simulink model "Quad_F450_Model"  (R2023a)
settings: Solver=FixedStepAuto  StartTime=0.0  StopTime=inf  FixedStep=Copter.SimTs  RelTol=1e-3
InitFcn:
  | load("motor_data.mat")
  | run("Parameters.m")
undefined symbols (not defined in the file or in its folder): Controller, Copter, DiscIntNeverNeededParam, Earth, init, Keyboard, motor_data, w_der_filt, WGS84
libraries: sharedutil x12, slpidlib x8, sharedtransform x5, aerolibpropulsionsys x4, simulink_extras x3, matrix_library x3, shared6dof x1, aerolibtransform2 x1, aerolibatmos2 x1, aerolibsim3d x1, sim3dlib x1
(part 3 of 3)

== system Quad_F450_Model/DYNAMIC_MODEL/Motor Forces and Moments/Motor 4/Moments ==
  rho : Inport
  w : Inport  Port=2
  Arm : Inport  Port=3
  Abs1 : Abs  SaturateOnIntegerOverflow=off
  Bus Selector : BusSelector  OutputSignals=prop4_cq,prop4_radius_m
  Constant : Constant  Value=pi
  Gain : Gain  Gain=-1
  Mxy : Constant  Value=[0 0]
  Product : Product  Inputs=5
  Product1 : Product
  Product5 : Product
  Product7 : Product
  Square : Math  Operator=square
  Vector Concatenate3 : Concatenate
  Mxyz : Outport
  wires:
  Product1/1 -> Product7/2
  Mxy/1 -> Vector Concatenate3/1
  rho/1 -> Product7/1
  Product7/1 -> Vector Concatenate3/2
  Abs1/1 -> Product5/2
  w/1 -> Abs1/1, Product5/1
  Vector Concatenate3/1 -> Mxyz/1
  [CQ] -> Product/1
  Constant/1 -> Product/2
  [R] -> Product/5, Square/1
  Square/1 -> Product/3, Product/4
  Product/1 -> Gain/1
  Product5/1 -> Product1/1
  Gain/1 -> [d_rads]
  [d_rads] -> Product1/2
  Arm/1 -> Bus Selector/1
  Bus Selector/1 -> [CQ]  "<prop4_cq>"
  Bus Selector/2 -> [R]  "<prop4_radius_m>"

== system Quad_F450_Model/DYNAMIC_MODEL/Motor Forces and Moments/Motor 4/Subsystem ==
  Vb : Inport
  pqr : Inport  Port=2
  w : Inport  Port=3
  Arm : Inport  Port=4
  3x3 Cross Product : sharedutil/3x3 Cross Product  aMode=aMode
  Add : Sum
  Bus Selector : BusSelector  OutputSignals=cg2motor_arm4_m
  Demux : Demux  Outputs=2
  Gain : Gain  Gain=Copter.blade_flap_active
  J : Subsystem
  Sum : aerolibpropulsionsys/Flap/Sum  Inputs=++|  CollapseDim=1  OutMin=[]  OutMax=[]  SampleTime=-1
  beta1 : Subsystem
  beta2 : Subsystem
  lc and mu : Subsystem
  a1s : Outport
  b1s : Outport  Port=2
  wires:
  w/1 -> beta2/2(w), beta1/4(w), lc and mu/2(w)
  Sum/1 -> lc and mu/1(Vr), J/1(Vr)  "Vr"
  Demux/1 -> a1s/1
  beta1/1(beta1) -> Add/1
  Add/1 -> Gain/1  "beta"
  pqr/1 -> beta2/3(pqr), 3x3 Cross Product/1
  beta2/1(beta2) -> Add/2
  Arm/1 -> Bus Selector/1, beta1/5(Arm), beta2/4(Arm), lc and mu/3(Arm)
  lc and mu/2(mu) -> beta2/1(mu), beta1/3(mu)
  lc and mu/1(lc) -> beta1/2(lc)
  Demux/2 -> b1s/1
  3x3 Cross Product/1 -> Sum/2
  Vb/1 -> Sum/1
  Bus Selector/1 -> 3x3 Cross Product/2  "<cg2motor_arm4_m>"
  J/1(J) -> beta1/1(J)
  Gain/1 -> Demux/1

== system Quad_F450_Model/DYNAMIC_MODEL/Motor Forces and Moments/Motor 1/Subsystem/J ==
  Vr : Inport
  Gain : Gain  Gain=-1
  Matrix Concatenate : Concatenate  Mode=Multidimensional array  ConcatenateDimension=2
  Selector2 : Selector  InputPortWidth=3  IndexOptions=Index vector (dialog)  Indices=[2]  OutputSizes=1
  Selector3 : Selector  InputPortWidth=3  IndexOptions=Index vector (dialog)  Indices=[1]  OutputSizes=1
  Trigonometric Function1 : Trigonometry  Operator=atan2
  Trigonometric Function2 : Trigonometry  Operator=sincos
  Vector Concatenate : Concatenate
  Vector Concatenate1 : Concatenate
  J : Outport
  wires:
  Vr/1 -> Selector2/1, Selector3/1
  Vector Concatenate/1 -> Matrix Concatenate/1
  Matrix Concatenate/1 -> J/1  "J"
  Trigonometric Function2/1 -> Gain/1, Vector Concatenate/2
  Trigonometric Function1/1 -> Trigonometric Function2/1  "j"
  Selector2/1 -> Trigonometric Function1/1
  Gain/1 -> Vector Concatenate1/1
  Selector3/1 -> Trigonometric Function1/2
  Trigonometric Function2/2 -> Vector Concatenate1/2, Vector Concatenate/1
  Vector Concatenate1/1 -> Matrix Concatenate/2

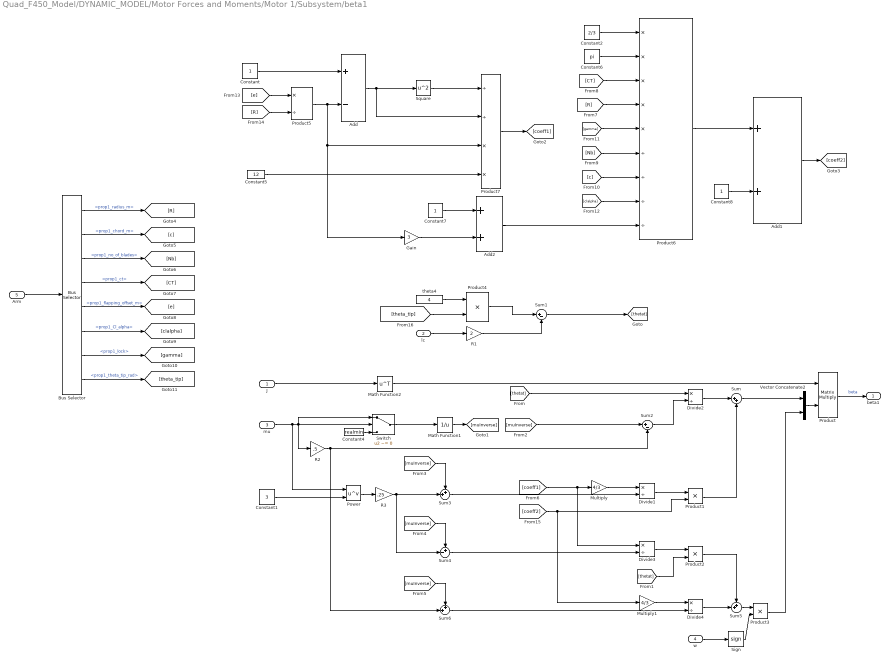
== system Quad_F450_Model/DYNAMIC_MODEL/Motor Forces and Moments/Motor 1/Subsystem/beta1 ==
  J : Inport
  lc : Inport  Port=2
  mu : Inport  Port=3
  w : Inport  Port=4
  Arm : Inport  Port=5
  Add : Sum  Inputs=+-
  Add1 : Sum
  Add2 : Sum
  Bus Selector : BusSelector  OutputSignals=prop1_radius_m,prop1_chord_m,prop1_no_of_blades,prop1_ct,prop1_flapping_offset_m,prop1_Cl_alpha,prop1_lock,prop1_theta_tip_rad
  Constant : Constant
  Constant1 : Constant  Value=3
  Constant2 : Constant  Value=2/3
  Constant4 : Constant  Value=realmin
  Constant5 : Constant  Value=12
  Constant6 : Constant  Value=pi
  Constant7 : Constant
  Constant8 : Constant
  Divide{1..4} (4 alike) : Product  Inputs=*/
  Gain : Gain  Gain=3
  Math Function1 : Math  Operator=reciprocal  SignedPower=on
  Math Function2 : Math  Operator=transpose  SignedPower=on
  Multiply : Gain  Gain=4/3
  Multiply1 : Gain  Gain=4/3
  Power : Math  Operator=pow
  Product : Product  Multiplication=Matrix(*)
  Product{1..4} (4 alike) : Product
  Product5 : Product  Inputs=*/
  Product6 : Product  Inputs=*****////
  Product7 : Product  Inputs=//**
  R1 : Gain  Gain=2
  R2 : Gain  Gain=.5
  R3 : Gain  Gain=.25
  Sign : Signum
  Square : Math  Operator=square
  Sum : Sum  Inputs=|++
  Sum1 : Sum  Inputs=|+-
  Sum2 : Sum  Inputs=|+-
  Sum3 : Sum  Inputs=++|
  Sum4 : Sum  Inputs=+-|
  Sum5 : Sum  Inputs=++|
  Sum6 : Sum  Inputs=++|
  Switch : Switch  Criteria=u2 ~= 0  SaturateOnIntegerOverflow=off  InputSameDT=off
  Vector Concatenate2 : Concatenate
  theta4 : Constant  Value=4
  beta1 : Outport
  wires:
  Sum6/1 -> Divide4/2
  Divide3/1 -> Product2/1
  Vector Concatenate2/1 -> Product/2
  mu/1 -> Power/1, R2/1, Switch/2, Switch/1
  R2/1 -> Sum6/2, Sum2/2
  [muInverse] -> Sum4/1
  R1/1 -> Sum1/2
  R3/1 -> Sum4/2, Sum3/2
  Math Function1/1 -> [muInverse]
  Product2/1 -> Sum5/1
  Multiply1/1 -> Divide4/1
  Product1/1 -> Sum/2
  Sum5/1 -> Product3/1
  [muInverse] -> Sum2/1
  Sum/1 -> Vector Concatenate2/1
  Multiply/1 -> Divide1/1
  Divide4/1 -> Sum5/2
  [muInverse] -> Sum6/1
  J/1 -> Math Function2/1
  [thetat] -> Product2/2
  Sum4/1 -> Divide3/2
  Product3/1 -> Vector Concatenate2/2
  [muInverse] -> Sum3/1
  Power/1 -> R3/1
  Switch/1 -> Math Function1/1
  Divide1/1 -> Product1/1
  [thetat] -> Divide2/1
  Constant4/1 -> Switch/3
  Sign/1 -> Product3/2
  Sum1/1 -> [thetat]
  lc/1 -> R1/1
  Product/1 -> beta1/1  "beta"
  w/1 -> Sign/1
  Sum2/1 -> Divide2/2
  Math Function2/1 -> Product/1
  Divide2/1 -> Sum/1
  Sum3/1 -> Divide1/2
  Constant1/1 -> Power/2
  Product4/1 -> Sum1/1
  theta4/1 -> Product4/1
  Square/1 -> Product7/1
  Add/1 -> Product7/2, Square/1
  Product5/1 -> Gain/1, Product7/3, Add/2
  [e] -> Product5/1
  [R] -> Product5/2
  Constant5/1 -> Product7/4
  Constant/1 -> Add/1
  Product7/1 -> [coeff1]
  [coeff1] -> Multiply/1, Divide3/1
  Constant2/1 -> Product6/1
  Constant6/1 -> Product6/2
  [CT] -> Product6/3
  [R] -> Product6/4
  [gamma] -> Product6/5
  [Nb] -> Product6/6
  [c] -> Product6/7
  [clalpha] -> Product6/8
  Constant7/1 -> Add2/1
  Gain/1 -> Add2/2
  Add2/1 -> Product6/9
  Product6/1 -> Add1/1
  Constant8/1 -> Add1/2
  Add1/1 -> [coeff2]
  [coeff2] -> Multiply1/1, Product1/2
  Arm/1 -> Bus Selector/1
  Bus Selector/1 -> [R]  "<prop1_radius_m>"
  Bus Selector/2 -> [c]  "<prop1_chord_m>"
  Bus Selector/3 -> [Nb]  "<prop1_no_of_blades>"
  Bus Selector/8 -> [theta_tip]  "<prop1_theta_tip_rad>"
  Bus Selector/7 -> [gamma]  "<prop1_lock>"
  Bus Selector/6 -> [clalpha]  "<prop1_Cl_alpha>"
  Bus Selector/5 -> [e]  "<prop1_flapping_offset_m>"
  Bus Selector/4 -> [CT]  "<prop1_ct>"
  [theta_tip] -> Product4/2

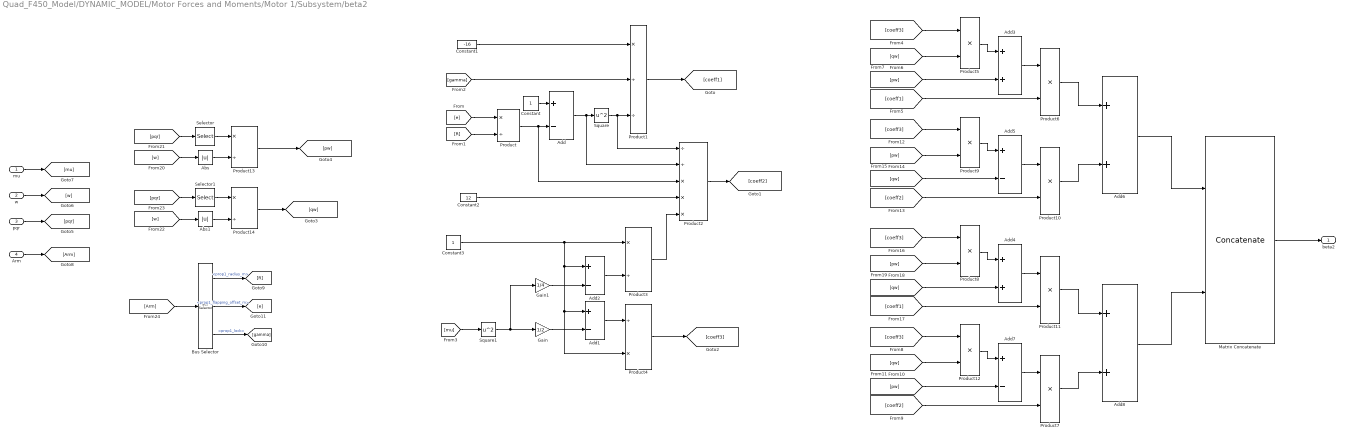
== system Quad_F450_Model/DYNAMIC_MODEL/Motor Forces and Moments/Motor 1/Subsystem/beta2 ==
  mu : Inport
  w : Inport  Port=2
  pqr : Inport  Port=3
  Arm : Inport  Port=4
  Abs : Abs  SaturateOnIntegerOverflow=off
  Abs1 : Abs  SaturateOnIntegerOverflow=off
  Add{,1..2,5,7} (5 alike) : Sum  Inputs=+-
  Add{3..4,6,8} (4 alike) : Sum
  Bus Selector : BusSelector  OutputSignals=prop1_radius_m,prop1_flapping_offset_m,prop1_lock
  Constant : Constant
  Constant1 : Constant  Value=-16
  Constant2 : Constant  Value=12
  Constant3 : Constant
  Gain : Gain  Gain=1/2
  Gain1 : Gain  Gain=1/4
  Matrix Concatenate : Concatenate  ConcatenateDimension=2
  Product{,3,13..14} (4 alike) : Product  Inputs=*/
  Product1 : Product  Inputs=*//
  Product{5..12} (8 alike) : Product
  Product2 : Product  Inputs=//***
  Product4 : Product  Inputs=/*
  Selector : Selector  InputPortWidth=3  IndexOptions=Index vector (dialog)  Indices=1  OutputSizes=1
  Selector1 : Selector  InputPortWidth=3  IndexOptions=Index vector (dialog)  Indices=1  OutputSizes=1
  Square : Math  Operator=square
  Square1 : Math  Operator=square
  beta2 : Outport
  wires:
  w/1 -> [w]
  mu/1 -> [mu]
  [e] -> Product/1
  [R] -> Product/2
  Constant/1 -> Add/1
  Product/1 -> Product2/3, Add/2
  Add/1 -> Product2/2, Square/1
  Square/1 -> Product2/1, Product1/3
  [gamma] -> Product1/2
  Constant1/1 -> Product1/1
  Constant2/1 -> Product2/4
  Constant3/1 -> Product4/2, Add1/1, Add2/1, Product3/1
  [mu] -> Square1/1
  Square1/1 -> Gain/1, Gain1/1
  Gain/1 -> Add1/2
  Gain1/1 -> Add2/2
  Add2/1 -> Product3/2
  Add1/1 -> Product4/1
  Product3/1 -> Product2/5
  Product1/1 -> [coeff1]
  Product2/1 -> [coeff2]
  Product4/1 -> [coeff3]
  [coeff3] -> Product5/1
  Product5/1 -> Add3/1
  Add3/1 -> Product6/1
  [coeff1] -> Product6/2
  [qw] -> Product5/2
  [pw] -> Add3/2
  Product6/1 -> Add6/1
  Product9/1 -> Add5/1
  [pw] -> Product9/2
  Add5/1 -> Product10/1
  [coeff2] -> Product10/2
  [qw] -> Add5/2
  [coeff3] -> Product9/1
  Product10/1 -> Add6/2
  Product12/1 -> Add7/1
  [coeff2] -> Product7/2
  [qw] -> Product12/2
  Add7/1 -> Product7/1
  Product8/1 -> Add4/1
  [coeff3] -> Product12/1
  [pw] -> Product8/2
  [pw] -> Add7/2
  Product7/1 -> Add8/2
  Add4/1 -> Product11/1
  [coeff1] -> Product11/2
  [qw] -> Add4/2
  [coeff3] -> Product8/1
  Product11/1 -> Add8/1
  Add6/1 -> Matrix Concatenate/1
  Add8/1 -> Matrix Concatenate/2
  pqr/1 -> [pqr]
  [pqr] -> Selector/1
  [w] -> Abs/1
  Selector/1 -> Product13/1
  Abs/1 -> Product13/2
  Product13/1 -> [pw]
  Abs1/1 -> Product14/2
  [w] -> Abs1/1
  Selector1/1 -> Product14/1
  Product14/1 -> [qw]
  [pqr] -> Selector1/1
  Arm/1 -> [Arm]
  [Arm] -> Bus Selector/1
  Matrix Concatenate/1 -> beta2/1
  Bus Selector/1 -> [R]  "<prop1_radius_m>"
  Bus Selector/2 -> [e]  "<prop1_flapping_offset_m>"
  Bus Selector/3 -> [gamma]  "<prop1_lock>"

== system Quad_F450_Model/DYNAMIC_MODEL/Motor Forces and Moments/Motor 1/Subsystem/lc and mu ==
  Vr : Inport
  w : Inport  Port=2
  Arm : Inport  Port=3
  Abs : Abs  SaturateOnIntegerOverflow=off
  Bus Selector : BusSelector  OutputSignals=prop1_radius_m
  Complex to Real-Imag : ComplexToRealImag  Output=Real
  Divide : Product  Inputs=*/
  Divide1 : Product  Inputs=*/
  Math Function : Math  Operator=square  SignedPower=on
  Product : Product
  Selector : Selector  InputPortWidth=3  IndexOptions=Index vector (dialog)  Indices=[1 2]  OutputSizes=1
  Selector1 : Selector  InputPortWidth=3  IndexOptions=Index vector (dialog)  Indices=[3]  OutputSizes=1
  Sqrt : Sqrt  OutputSignalType=complex
  Sum of Elements : Sum  Inputs=+
  lc : Outport
  mu : Outport  Port=2
  wires:
  Selector/1 -> Math Function/1
  Sqrt/1 -> Complex to Real-Imag/1
  Math Function/1 -> Sum of Elements/1
  w/1 -> Abs/1
  Selector1/1 -> Divide1/1
  Product/1 -> Divide/2, Divide1/2
  Divide1/1 -> lc/1  "lc"
  Vr/1 -> Selector/1, Selector1/1
  Sum of Elements/1 -> Sqrt/1
  Divide/1 -> mu/1  "mu"
  Complex to Real-Imag/1 -> Divide/1
  Abs/1 -> Product/1
  Arm/1 -> Bus Selector/1  "r"
  Bus Selector/1 -> Product/2  "<prop1_radius_m>"

== system Quad_F450_Model/DYNAMIC_MODEL/Motor Forces and Moments/Motor 2/Subsystem/J ==
  Vr : Inport
  Gain : Gain  Gain=-1
  Matrix Concatenate : Concatenate  Mode=Multidimensional array  ConcatenateDimension=2
  Selector2 : Selector  InputPortWidth=3  IndexOptions=Index vector (dialog)  Indices=[2]  OutputSizes=1
  Selector3 : Selector  InputPortWidth=3  IndexOptions=Index vector (dialog)  Indices=[1]  OutputSizes=1
  Trigonometric Function1 : Trigonometry  Operator=atan2
  Trigonometric Function2 : Trigonometry  Operator=sincos
  Vector Concatenate : Concatenate
  Vector Concatenate1 : Concatenate
  J : Outport
  wires:
  Vr/1 -> Selector2/1, Selector3/1
  Vector Concatenate/1 -> Matrix Concatenate/1
  Matrix Concatenate/1 -> J/1  "J"
  Trigonometric Function2/1 -> Gain/1, Vector Concatenate/2
  Trigonometric Function1/1 -> Trigonometric Function2/1  "j"
  Selector2/1 -> Trigonometric Function1/1
  Gain/1 -> Vector Concatenate1/1
  Selector3/1 -> Trigonometric Function1/2
  Trigonometric Function2/2 -> Vector Concatenate1/2, Vector Concatenate/1
  Vector Concatenate1/1 -> Matrix Concatenate/2

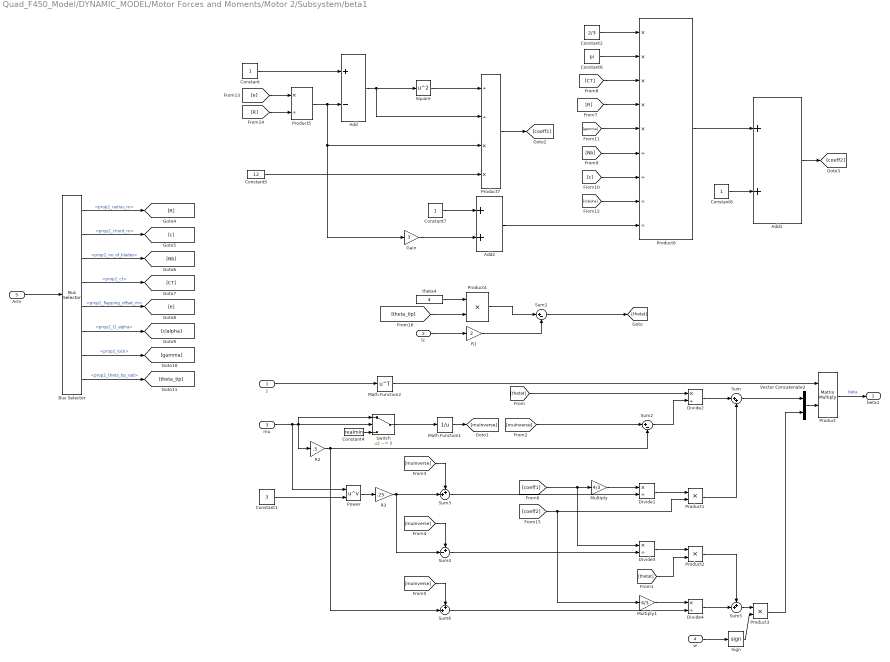
== system Quad_F450_Model/DYNAMIC_MODEL/Motor Forces and Moments/Motor 2/Subsystem/beta1 ==
  J : Inport
  lc : Inport  Port=2
  mu : Inport  Port=3
  w : Inport  Port=4
  Arm : Inport  Port=5
  Add : Sum  Inputs=+-
  Add1 : Sum
  Add2 : Sum
  Bus Selector : BusSelector  OutputSignals=prop2_radius_m,prop2_chord_m,prop2_no_of_blades,prop2_ct,prop2_flapping_offset_m,prop2_Cl_alpha,prop2_lock,prop2_theta_tip_rad
  Constant : Constant
  Constant1 : Constant  Value=3
  Constant2 : Constant  Value=2/3
  Constant4 : Constant  Value=realmin
  Constant5 : Constant  Value=12
  Constant6 : Constant  Value=pi
  Constant7 : Constant
  Constant8 : Constant
  Divide{1..4} (4 alike) : Product  Inputs=*/
  Gain : Gain  Gain=3
  Math Function1 : Math  Operator=reciprocal  SignedPower=on
  Math Function2 : Math  Operator=transpose  SignedPower=on
  Multiply : Gain  Gain=4/3
  Multiply1 : Gain  Gain=4/3
  Power : Math  Operator=pow
  Product : Product  Multiplication=Matrix(*)
  Product{1..4} (4 alike) : Product
  Product5 : Product  Inputs=*/
  Product6 : Product  Inputs=*****////
  Product7 : Product  Inputs=//**
  R1 : Gain  Gain=2
  R2 : Gain  Gain=.5
  R3 : Gain  Gain=.25
  Sign : Signum
  Square : Math  Operator=square
  Sum : Sum  Inputs=|++
  Sum1 : Sum  Inputs=|+-
  Sum2 : Sum  Inputs=|+-
  Sum3 : Sum  Inputs=++|
  Sum4 : Sum  Inputs=+-|
  Sum5 : Sum  Inputs=++|
  Sum6 : Sum  Inputs=++|
  Switch : Switch  Criteria=u2 ~= 0  SaturateOnIntegerOverflow=off  InputSameDT=off
  Vector Concatenate2 : Concatenate
  theta4 : Constant  Value=4
  beta1 : Outport
  wires:
  Sum6/1 -> Divide4/2
  Divide3/1 -> Product2/1
  Vector Concatenate2/1 -> Product/2
  mu/1 -> Power/1, R2/1, Switch/2, Switch/1
  R2/1 -> Sum6/2, Sum2/2
  [muInverse] -> Sum4/1
  R1/1 -> Sum1/2
  R3/1 -> Sum4/2, Sum3/2
  Math Function1/1 -> [muInverse]
  Product2/1 -> Sum5/1
  Multiply1/1 -> Divide4/1
  Product1/1 -> Sum/2
  Sum5/1 -> Product3/1
  [muInverse] -> Sum2/1
  Sum/1 -> Vector Concatenate2/1
  Multiply/1 -> Divide1/1
  Divide4/1 -> Sum5/2
  [muInverse] -> Sum6/1
  J/1 -> Math Function2/1
  [thetat] -> Product2/2
  Sum4/1 -> Divide3/2
  Product3/1 -> Vector Concatenate2/2
  [muInverse] -> Sum3/1
  Power/1 -> R3/1
  Switch/1 -> Math Function1/1
  Divide1/1 -> Product1/1
  [thetat] -> Divide2/1
  Constant4/1 -> Switch/3
  Sign/1 -> Product3/2
  Sum1/1 -> [thetat]
  lc/1 -> R1/1
  Product/1 -> beta1/1  "beta"
  w/1 -> Sign/1
  Sum2/1 -> Divide2/2
  Math Function2/1 -> Product/1
  Divide2/1 -> Sum/1
  Sum3/1 -> Divide1/2
  Constant1/1 -> Power/2
  Product4/1 -> Sum1/1
  theta4/1 -> Product4/1
  Square/1 -> Product7/1
  Add/1 -> Product7/2, Square/1
  Product5/1 -> Gain/1, Product7/3, Add/2
  [e] -> Product5/1
  [R] -> Product5/2
  Constant5/1 -> Product7/4
  Constant/1 -> Add/1
  Product7/1 -> [coeff1]
  [coeff1] -> Multiply/1, Divide3/1
  Constant2/1 -> Product6/1
  Constant6/1 -> Product6/2
  [CT] -> Product6/3
  [R] -> Product6/4
  [gamma] -> Product6/5
  [Nb] -> Product6/6
  [c] -> Product6/7
  [clalpha] -> Product6/8
  Constant7/1 -> Add2/1
  Gain/1 -> Add2/2
  Add2/1 -> Product6/9
  Product6/1 -> Add1/1
  Constant8/1 -> Add1/2
  Add1/1 -> [coeff2]
  [coeff2] -> Multiply1/1, Product1/2
  Arm/1 -> Bus Selector/1
  Bus Selector/1 -> [R]  "<prop2_radius_m>"
  Bus Selector/2 -> [c]  "<prop2_chord_m>"
  Bus Selector/3 -> [Nb]  "<prop2_no_of_blades>"
  Bus Selector/8 -> [theta_tip]  "<prop2_theta_tip_rad>"
  Bus Selector/7 -> [gamma]  "<prop2_lock>"
  Bus Selector/6 -> [clalpha]  "<prop2_Cl_alpha>"
  Bus Selector/5 -> [e]  "<prop2_flapping_offset_m>"
  Bus Selector/4 -> [CT]  "<prop2_ct>"
  [theta_tip] -> Product4/2

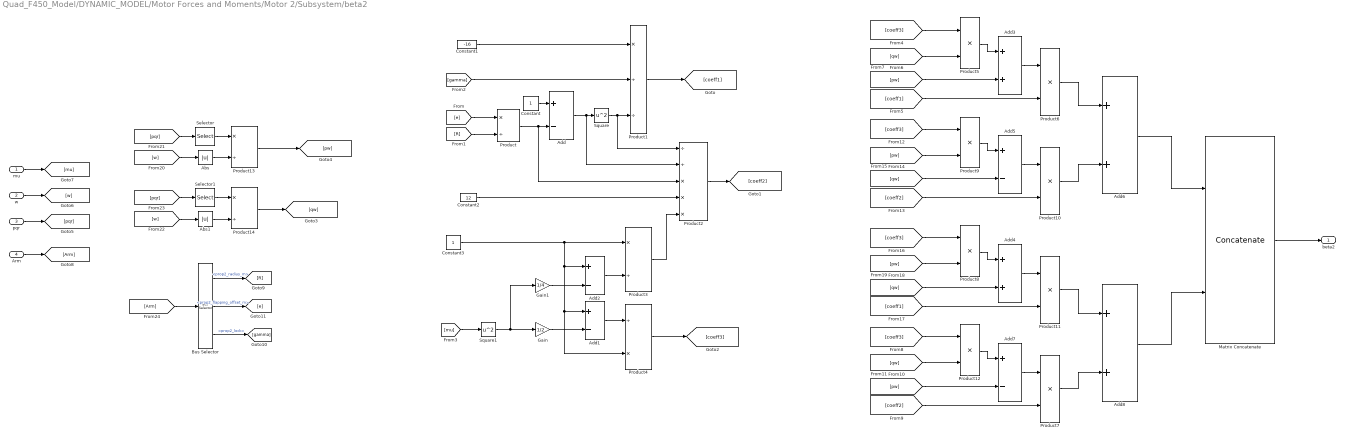
== system Quad_F450_Model/DYNAMIC_MODEL/Motor Forces and Moments/Motor 2/Subsystem/beta2 ==
  mu : Inport
  w : Inport  Port=2
  pqr : Inport  Port=3
  Arm : Inport  Port=4
  Abs : Abs  SaturateOnIntegerOverflow=off
  Abs1 : Abs  SaturateOnIntegerOverflow=off
  Add{,1..2,5,7} (5 alike) : Sum  Inputs=+-
  Add{3..4,6,8} (4 alike) : Sum
  Bus Selector : BusSelector  OutputSignals=prop2_radius_m,prop2_flapping_offset_m,prop2_lock
  Constant : Constant
  Constant1 : Constant  Value=-16
  Constant2 : Constant  Value=12
  Constant3 : Constant
  Gain : Gain  Gain=1/2
  Gain1 : Gain  Gain=1/4
  Matrix Concatenate : Concatenate  ConcatenateDimension=2
  Product{,3,13..14} (4 alike) : Product  Inputs=*/
  Product1 : Product  Inputs=*//
  Product{5..12} (8 alike) : Product
  Product2 : Product  Inputs=//***
  Product4 : Product  Inputs=/*
  Selector : Selector  InputPortWidth=3  IndexOptions=Index vector (dialog)  Indices=1  OutputSizes=1
  Selector1 : Selector  InputPortWidth=3  IndexOptions=Index vector (dialog)  Indices=1  OutputSizes=1
  Square : Math  Operator=square
  Square1 : Math  Operator=square
  beta2 : Outport
  wires:
  w/1 -> [w]
  mu/1 -> [mu]
  [e] -> Product/1
  [R] -> Product/2
  Constant/1 -> Add/1
  Product/1 -> Product2/3, Add/2
  Add/1 -> Product2/2, Square/1
  Square/1 -> Product2/1, Product1/3
  [gamma] -> Product1/2
  Constant1/1 -> Product1/1
  Constant2/1 -> Product2/4
  Constant3/1 -> Product4/2, Add1/1, Add2/1, Product3/1
  [mu] -> Square1/1
  Square1/1 -> Gain/1, Gain1/1
  Gain/1 -> Add1/2
  Gain1/1 -> Add2/2
  Add2/1 -> Product3/2
  Add1/1 -> Product4/1
  Product3/1 -> Product2/5
  Product1/1 -> [coeff1]
  Product2/1 -> [coeff2]
  Product4/1 -> [coeff3]
  [coeff3] -> Product5/1
  Product5/1 -> Add3/1
  Add3/1 -> Product6/1
  [coeff1] -> Product6/2
  [qw] -> Product5/2
  [pw] -> Add3/2
  Product6/1 -> Add6/1
  Product9/1 -> Add5/1
  [pw] -> Product9/2
  Add5/1 -> Product10/1
  [coeff2] -> Product10/2
  [qw] -> Add5/2
  [coeff3] -> Product9/1
  Product10/1 -> Add6/2
  Product12/1 -> Add7/1
  [coeff2] -> Product7/2
  [qw] -> Product12/2
  Add7/1 -> Product7/1
  Product8/1 -> Add4/1
  [coeff3] -> Product12/1
  [pw] -> Product8/2
  [pw] -> Add7/2
  Product7/1 -> Add8/2
  Add4/1 -> Product11/1
  [coeff1] -> Product11/2
  [qw] -> Add4/2
  [coeff3] -> Product8/1
  Product11/1 -> Add8/1
  Add6/1 -> Matrix Concatenate/1
  Add8/1 -> Matrix Concatenate/2
  pqr/1 -> [pqr]
  [pqr] -> Selector/1
  [w] -> Abs/1
  Selector/1 -> Product13/1
  Abs/1 -> Product13/2
  Product13/1 -> [pw]
  Abs1/1 -> Product14/2
  [w] -> Abs1/1
  Selector1/1 -> Product14/1
  Product14/1 -> [qw]
  [pqr] -> Selector1/1
  Arm/1 -> [Arm]
  [Arm] -> Bus Selector/1
  Matrix Concatenate/1 -> beta2/1
  Bus Selector/1 -> [R]  "<prop2_radius_m>"
  Bus Selector/2 -> [e]  "<prop2_flapping_offset_m>"
  Bus Selector/3 -> [gamma]  "<prop2_lock>"

== system Quad_F450_Model/DYNAMIC_MODEL/Motor Forces and Moments/Motor 2/Subsystem/lc and mu ==
  Vr : Inport
  w : Inport  Port=2
  Arm : Inport  Port=3
  Abs : Abs  SaturateOnIntegerOverflow=off
  Bus Selector : BusSelector  OutputSignals=prop2_radius_m
  Complex to Real-Imag : ComplexToRealImag  Output=Real
  Divide : Product  Inputs=*/
  Divide1 : Product  Inputs=*/
  Math Function : Math  Operator=square  SignedPower=on
  Product : Product
  Selector : Selector  InputPortWidth=3  IndexOptions=Index vector (dialog)  Indices=[1 2]  OutputSizes=1
  Selector1 : Selector  InputPortWidth=3  IndexOptions=Index vector (dialog)  Indices=[3]  OutputSizes=1
  Sqrt : Sqrt  OutputSignalType=complex
  Sum of Elements : Sum  Inputs=+
  lc : Outport
  mu : Outport  Port=2
  wires:
  Selector/1 -> Math Function/1
  Sqrt/1 -> Complex to Real-Imag/1
  Math Function/1 -> Sum of Elements/1
  w/1 -> Abs/1
  Selector1/1 -> Divide1/1
  Product/1 -> Divide/2, Divide1/2
  Divide1/1 -> lc/1  "lc"
  Vr/1 -> Selector/1, Selector1/1
  Sum of Elements/1 -> Sqrt/1
  Divide/1 -> mu/1  "mu"
  Complex to Real-Imag/1 -> Divide/1
  Abs/1 -> Product/1
  Arm/1 -> Bus Selector/1  "r"
  Bus Selector/1 -> Product/2  "<prop2_radius_m>"

== system Quad_F450_Model/DYNAMIC_MODEL/Motor Forces and Moments/Motor 3/Subsystem/J ==
  Vr : Inport
  Gain : Gain  Gain=-1
  Matrix Concatenate : Concatenate  Mode=Multidimensional array  ConcatenateDimension=2
  Selector2 : Selector  InputPortWidth=3  IndexOptions=Index vector (dialog)  Indices=[2]  OutputSizes=1
  Selector3 : Selector  InputPortWidth=3  IndexOptions=Index vector (dialog)  Indices=[1]  OutputSizes=1
  Trigonometric Function1 : Trigonometry  Operator=atan2
  Trigonometric Function2 : Trigonometry  Operator=sincos
  Vector Concatenate : Concatenate
  Vector Concatenate1 : Concatenate
  J : Outport
  wires:
  Vr/1 -> Selector2/1, Selector3/1
  Vector Concatenate/1 -> Matrix Concatenate/1
  Matrix Concatenate/1 -> J/1  "J"
  Trigonometric Function2/1 -> Gain/1, Vector Concatenate/2
  Trigonometric Function1/1 -> Trigonometric Function2/1  "j"
  Selector2/1 -> Trigonometric Function1/1
  Gain/1 -> Vector Concatenate1/1
  Selector3/1 -> Trigonometric Function1/2
  Trigonometric Function2/2 -> Vector Concatenate1/2, Vector Concatenate/1
  Vector Concatenate1/1 -> Matrix Concatenate/2

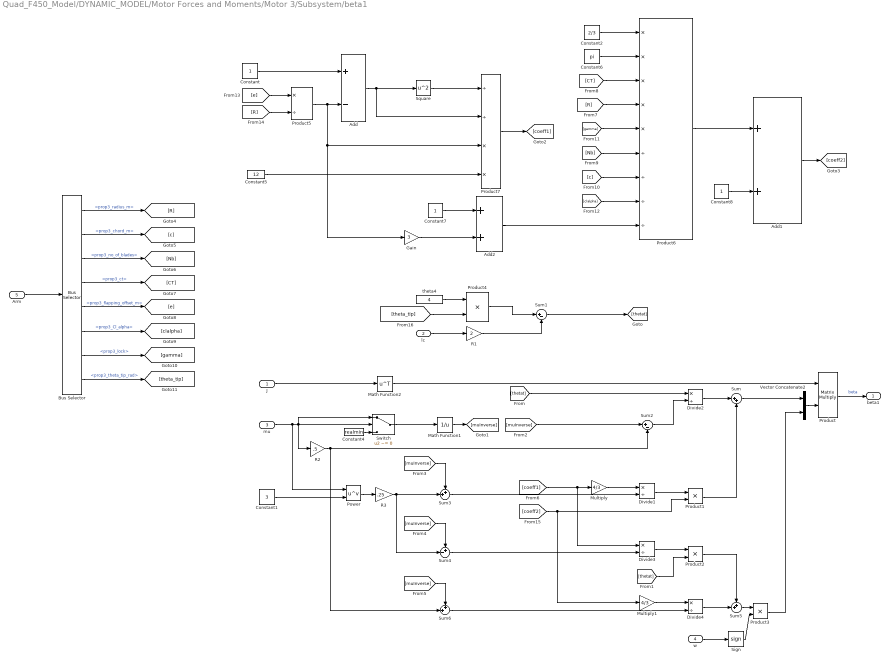
== system Quad_F450_Model/DYNAMIC_MODEL/Motor Forces and Moments/Motor 3/Subsystem/beta1 ==
  J : Inport
  lc : Inport  Port=2
  mu : Inport  Port=3
  w : Inport  Port=4
  Arm : Inport  Port=5
  Add : Sum  Inputs=+-
  Add1 : Sum
  Add2 : Sum
  Bus Selector : BusSelector  OutputSignals=prop3_radius_m,prop3_chord_m,prop3_no_of_blades,prop3_ct,prop3_flapping_offset_m,prop3_Cl_alpha,prop3_lock,prop3_theta_tip_rad
  Constant : Constant
  Constant1 : Constant  Value=3
  Constant2 : Constant  Value=2/3
  Constant4 : Constant  Value=realmin
  Constant5 : Constant  Value=12
  Constant6 : Constant  Value=pi
  Constant7 : Constant
  Constant8 : Constant
  Divide{1..4} (4 alike) : Product  Inputs=*/
  Gain : Gain  Gain=3
  Math Function1 : Math  Operator=reciprocal  SignedPower=on
  Math Function2 : Math  Operator=transpose  SignedPower=on
  Multiply : Gain  Gain=4/3
  Multiply1 : Gain  Gain=4/3
  Power : Math  Operator=pow
  Product : Product  Multiplication=Matrix(*)
  Product{1..4} (4 alike) : Product
  Product5 : Product  Inputs=*/
  Product6 : Product  Inputs=*****////
  Product7 : Product  Inputs=//**
  R1 : Gain  Gain=2
  R2 : Gain  Gain=.5
  R3 : Gain  Gain=.25
  Sign : Signum
  Square : Math  Operator=square
  Sum : Sum  Inputs=|++
  Sum1 : Sum  Inputs=|+-
  Sum2 : Sum  Inputs=|+-
  Sum3 : Sum  Inputs=++|
  Sum4 : Sum  Inputs=+-|
  Sum5 : Sum  Inputs=++|
  Sum6 : Sum  Inputs=++|
  Switch : Switch  Criteria=u2 ~= 0  SaturateOnIntegerOverflow=off  InputSameDT=off
  Vector Concatenate2 : Concatenate
  theta4 : Constant  Value=4
  beta1 : Outport
  wires:
  Sum6/1 -> Divide4/2
  Divide3/1 -> Product2/1
  Vector Concatenate2/1 -> Product/2
  mu/1 -> Power/1, R2/1, Switch/2, Switch/1
  R2/1 -> Sum6/2, Sum2/2
  [muInverse] -> Sum4/1
  R1/1 -> Sum1/2
  R3/1 -> Sum4/2, Sum3/2
  Math Function1/1 -> [muInverse]
  Product2/1 -> Sum5/1
  Multiply1/1 -> Divide4/1
  Product1/1 -> Sum/2
  Sum5/1 -> Product3/1
  [muInverse] -> Sum2/1
  Sum/1 -> Vector Concatenate2/1
  Multiply/1 -> Divide1/1
  Divide4/1 -> Sum5/2
  [muInverse] -> Sum6/1
  J/1 -> Math Function2/1
  [thetat] -> Product2/2
  Sum4/1 -> Divide3/2
  Product3/1 -> Vector Concatenate2/2
  [muInverse] -> Sum3/1
  Power/1 -> R3/1
  Switch/1 -> Math Function1/1
  Divide1/1 -> Product1/1
  [thetat] -> Divide2/1
  Constant4/1 -> Switch/3
  Sign/1 -> Product3/2
  Sum1/1 -> [thetat]
  lc/1 -> R1/1
  Product/1 -> beta1/1  "beta"
  w/1 -> Sign/1
  Sum2/1 -> Divide2/2
  Math Function2/1 -> Product/1
  Divide2/1 -> Sum/1
  Sum3/1 -> Divide1/2
  Constant1/1 -> Power/2
  Product4/1 -> Sum1/1
  theta4/1 -> Product4/1
  Square/1 -> Product7/1
  Add/1 -> Product7/2, Square/1
  Product5/1 -> Gain/1, Product7/3, Add/2
  [e] -> Product5/1
  [R] -> Product5/2
  Constant5/1 -> Product7/4
  Constant/1 -> Add/1
  Product7/1 -> [coeff1]
  [coeff1] -> Multiply/1, Divide3/1
  Constant2/1 -> Product6/1
  Constant6/1 -> Product6/2
  [CT] -> Product6/3
  [R] -> Product6/4
  [gamma] -> Product6/5
  [Nb] -> Product6/6
  [c] -> Product6/7
  [clalpha] -> Product6/8
  Constant7/1 -> Add2/1
  Gain/1 -> Add2/2
  Add2/1 -> Product6/9
  Product6/1 -> Add1/1
  Constant8/1 -> Add1/2
  Add1/1 -> [coeff2]
  [coeff2] -> Multiply1/1, Product1/2
  Arm/1 -> Bus Selector/1
  Bus Selector/1 -> [R]  "<prop3_radius_m>"
  Bus Selector/2 -> [c]  "<prop3_chord_m>"
  Bus Selector/3 -> [Nb]  "<prop3_no_of_blades>"
  Bus Selector/8 -> [theta_tip]  "<prop3_theta_tip_rad>"
  Bus Selector/7 -> [gamma]  "<prop3_lock>"
  Bus Selector/6 -> [clalpha]  "<prop3_Cl_alpha>"
  Bus Selector/5 -> [e]  "<prop3_flapping_offset_m>"
  Bus Selector/4 -> [CT]  "<prop3_ct>"
  [theta_tip] -> Product4/2

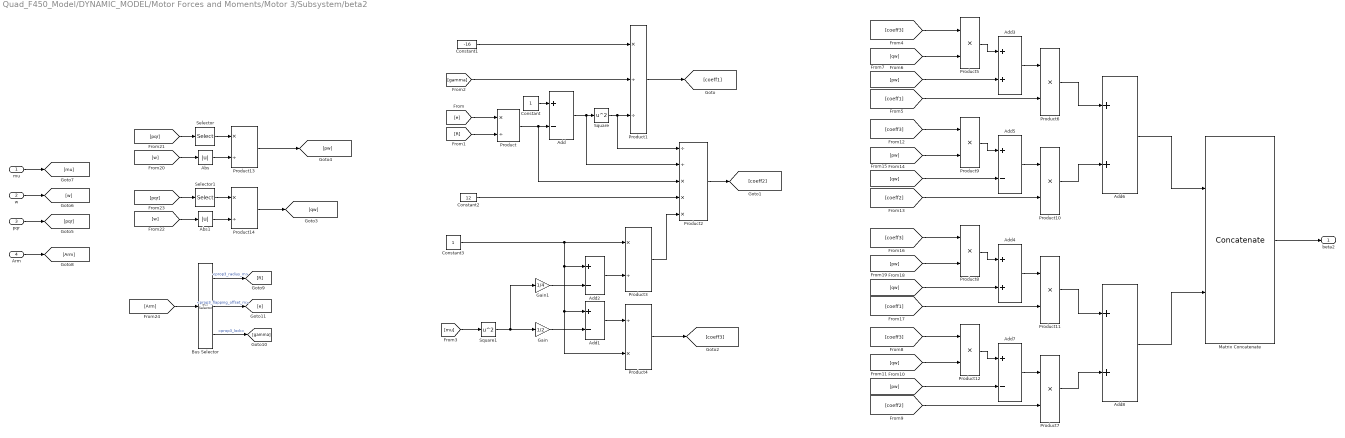
== system Quad_F450_Model/DYNAMIC_MODEL/Motor Forces and Moments/Motor 3/Subsystem/beta2 ==
  mu : Inport
  w : Inport  Port=2
  pqr : Inport  Port=3
  Arm : Inport  Port=4
  Abs : Abs  SaturateOnIntegerOverflow=off
  Abs1 : Abs  SaturateOnIntegerOverflow=off
  Add{,1..2,5,7} (5 alike) : Sum  Inputs=+-
  Add{3..4,6,8} (4 alike) : Sum
  Bus Selector : BusSelector  OutputSignals=prop3_radius_m,prop3_flapping_offset_m,prop3_lock
  Constant : Constant
  Constant1 : Constant  Value=-16
  Constant2 : Constant  Value=12
  Constant3 : Constant
  Gain : Gain  Gain=1/2
  Gain1 : Gain  Gain=1/4
  Matrix Concatenate : Concatenate  ConcatenateDimension=2
  Product{,3,13..14} (4 alike) : Product  Inputs=*/
  Product1 : Product  Inputs=*//
  Product{5..12} (8 alike) : Product
  Product2 : Product  Inputs=//***
  Product4 : Product  Inputs=/*
  Selector : Selector  InputPortWidth=3  IndexOptions=Index vector (dialog)  Indices=1  OutputSizes=1
  Selector1 : Selector  InputPortWidth=3  IndexOptions=Index vector (dialog)  Indices=1  OutputSizes=1
  Square : Math  Operator=square
  Square1 : Math  Operator=square
  beta2 : Outport
  wires:
  w/1 -> [w]
  mu/1 -> [mu]
  [e] -> Product/1
  [R] -> Product/2
  Constant/1 -> Add/1
  Product/1 -> Product2/3, Add/2
  Add/1 -> Product2/2, Square/1
  Square/1 -> Product2/1, Product1/3
  [gamma] -> Product1/2
  Constant1/1 -> Product1/1
  Constant2/1 -> Product2/4
  Constant3/1 -> Product4/2, Add1/1, Add2/1, Product3/1
  [mu] -> Square1/1
  Square1/1 -> Gain/1, Gain1/1
  Gain/1 -> Add1/2
  Gain1/1 -> Add2/2
  Add2/1 -> Product3/2
  Add1/1 -> Product4/1
  Product3/1 -> Product2/5
  Product1/1 -> [coeff1]
  Product2/1 -> [coeff2]
  Product4/1 -> [coeff3]
  [coeff3] -> Product5/1
  Product5/1 -> Add3/1
  Add3/1 -> Product6/1
  [coeff1] -> Product6/2
  [qw] -> Product5/2
  [pw] -> Add3/2
  Product6/1 -> Add6/1
  Product9/1 -> Add5/1
  [pw] -> Product9/2
  Add5/1 -> Product10/1
  [coeff2] -> Product10/2
  [qw] -> Add5/2
  [coeff3] -> Product9/1
  Product10/1 -> Add6/2
  Product12/1 -> Add7/1
  [coeff2] -> Product7/2
  [qw] -> Product12/2
  Add7/1 -> Product7/1
  Product8/1 -> Add4/1
  [coeff3] -> Product12/1
  [pw] -> Product8/2
  [pw] -> Add7/2
  Product7/1 -> Add8/2
  Add4/1 -> Product11/1
  [coeff1] -> Product11/2
  [qw] -> Add4/2
  [coeff3] -> Product8/1
  Product11/1 -> Add8/1
  Add6/1 -> Matrix Concatenate/1
  Add8/1 -> Matrix Concatenate/2
  pqr/1 -> [pqr]
  [pqr] -> Selector/1
  [w] -> Abs/1
  Selector/1 -> Product13/1
  Abs/1 -> Product13/2
  Product13/1 -> [pw]
  Abs1/1 -> Product14/2
  [w] -> Abs1/1
  Selector1/1 -> Product14/1
  Product14/1 -> [qw]
  [pqr] -> Selector1/1
  Arm/1 -> [Arm]
  [Arm] -> Bus Selector/1
  Matrix Concatenate/1 -> beta2/1
  Bus Selector/1 -> [R]  "<prop3_radius_m>"
  Bus Selector/2 -> [e]  "<prop3_flapping_offset_m>"
  Bus Selector/3 -> [gamma]  "<prop3_lock>"

== system Quad_F450_Model/DYNAMIC_MODEL/Motor Forces and Moments/Motor 3/Subsystem/lc and mu ==
  Vr : Inport
  w : Inport  Port=2
  Arm : Inport  Port=3
  Abs : Abs  SaturateOnIntegerOverflow=off
  Bus Selector : BusSelector  OutputSignals=prop3_radius_m
  Complex to Real-Imag : ComplexToRealImag  Output=Real
  Divide : Product  Inputs=*/
  Divide1 : Product  Inputs=*/
  Math Function : Math  Operator=square  SignedPower=on
  Product : Product
  Selector : Selector  InputPortWidth=3  IndexOptions=Index vector (dialog)  Indices=[1 2]  OutputSizes=1
  Selector1 : Selector  InputPortWidth=3  IndexOptions=Index vector (dialog)  Indices=[3]  OutputSizes=1
  Sqrt : Sqrt  OutputSignalType=complex
  Sum of Elements : Sum  Inputs=+
  lc : Outport
  mu : Outport  Port=2
  wires:
  Selector/1 -> Math Function/1
  Sqrt/1 -> Complex to Real-Imag/1
  Math Function/1 -> Sum of Elements/1
  w/1 -> Abs/1
  Selector1/1 -> Divide1/1
  Product/1 -> Divide/2, Divide1/2
  Divide1/1 -> lc/1  "lc"
  Vr/1 -> Selector/1, Selector1/1
  Sum of Elements/1 -> Sqrt/1
  Divide/1 -> mu/1  "mu"
  Complex to Real-Imag/1 -> Divide/1
  Abs/1 -> Product/1
  Arm/1 -> Bus Selector/1  "r"
  Bus Selector/1 -> Product/2  "<prop3_radius_m>"

== system Quad_F450_Model/DYNAMIC_MODEL/Motor Forces and Moments/Motor 4/Subsystem/J ==
  Vr : Inport
  Gain : Gain  Gain=-1
  Matrix Concatenate : Concatenate  Mode=Multidimensional array  ConcatenateDimension=2
  Selector2 : Selector  InputPortWidth=3  IndexOptions=Index vector (dialog)  Indices=[2]  OutputSizes=1
  Selector3 : Selector  InputPortWidth=3  IndexOptions=Index vector (dialog)  Indices=[1]  OutputSizes=1
  Trigonometric Function1 : Trigonometry  Operator=atan2
  Trigonometric Function2 : Trigonometry  Operator=sincos
  Vector Concatenate : Concatenate
  Vector Concatenate1 : Concatenate
  J : Outport
  wires:
  Vr/1 -> Selector2/1, Selector3/1
  Vector Concatenate/1 -> Matrix Concatenate/1
  Matrix Concatenate/1 -> J/1  "J"
  Trigonometric Function2/1 -> Gain/1, Vector Concatenate/2
  Trigonometric Function1/1 -> Trigonometric Function2/1  "j"
  Selector2/1 -> Trigonometric Function1/1
  Gain/1 -> Vector Concatenate1/1
  Selector3/1 -> Trigonometric Function1/2
  Trigonometric Function2/2 -> Vector Concatenate1/2, Vector Concatenate/1
  Vector Concatenate1/1 -> Matrix Concatenate/2

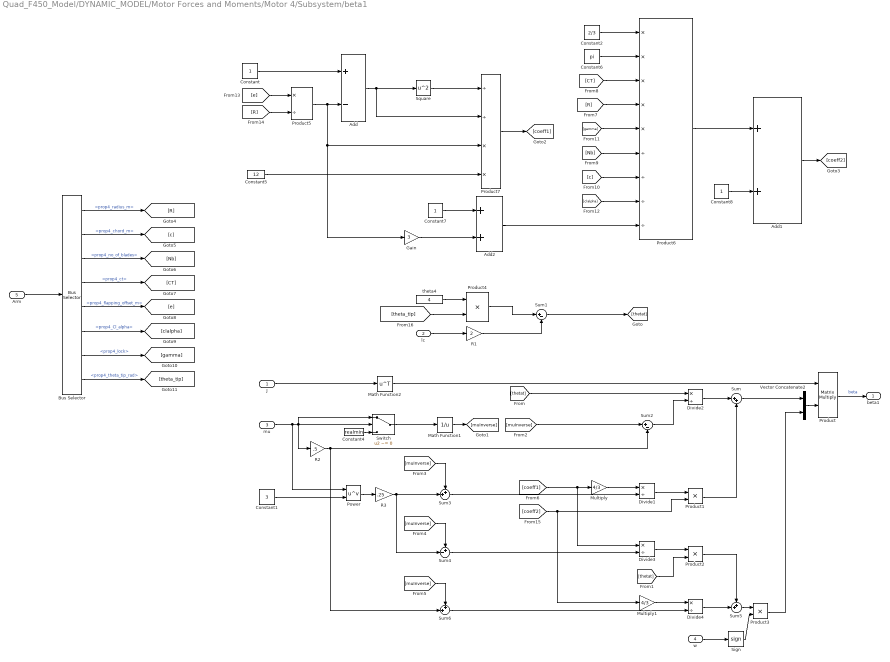
== system Quad_F450_Model/DYNAMIC_MODEL/Motor Forces and Moments/Motor 4/Subsystem/beta1 ==
  J : Inport
  lc : Inport  Port=2
  mu : Inport  Port=3
  w : Inport  Port=4
  Arm : Inport  Port=5
  Add : Sum  Inputs=+-
  Add1 : Sum
  Add2 : Sum
  Bus Selector : BusSelector  OutputSignals=prop4_radius_m,prop4_chord_m,prop4_no_of_blades,prop4_ct,prop4_flapping_offset_m,prop4_Cl_alpha,prop4_lock,prop4_theta_tip_rad
  Constant : Constant
  Constant1 : Constant  Value=3
  Constant2 : Constant  Value=2/3
  Constant4 : Constant  Value=realmin
  Constant5 : Constant  Value=12
  Constant6 : Constant  Value=pi
  Constant7 : Constant
  Constant8 : Constant
  Divide{1..4} (4 alike) : Product  Inputs=*/
  Gain : Gain  Gain=3
  Math Function1 : Math  Operator=reciprocal  SignedPower=on
  Math Function2 : Math  Operator=transpose  SignedPower=on
  Multiply : Gain  Gain=4/3
  Multiply1 : Gain  Gain=4/3
  Power : Math  Operator=pow
  Product : Product  Multiplication=Matrix(*)
  Product{1..4} (4 alike) : Product
  Product5 : Product  Inputs=*/
  Product6 : Product  Inputs=*****////
  Product7 : Product  Inputs=//**
  R1 : Gain  Gain=2
  R2 : Gain  Gain=.5
  R3 : Gain  Gain=.25
  Sign : Signum
  Square : Math  Operator=square
  Sum : Sum  Inputs=|++
  Sum1 : Sum  Inputs=|+-
  Sum2 : Sum  Inputs=|+-
  Sum3 : Sum  Inputs=++|
  Sum4 : Sum  Inputs=+-|
  Sum5 : Sum  Inputs=++|
  Sum6 : Sum  Inputs=++|
  Switch : Switch  Criteria=u2 ~= 0  SaturateOnIntegerOverflow=off  InputSameDT=off
  Vector Concatenate2 : Concatenate
  theta4 : Constant  Value=4
  beta1 : Outport
  wires:
  Sum6/1 -> Divide4/2
  Divide3/1 -> Product2/1
  Vector Concatenate2/1 -> Product/2
  mu/1 -> Power/1, R2/1, Switch/2, Switch/1
  R2/1 -> Sum6/2, Sum2/2
  [muInverse] -> Sum4/1
  R1/1 -> Sum1/2
  R3/1 -> Sum4/2, Sum3/2
  Math Function1/1 -> [muInverse]
  Product2/1 -> Sum5/1
  Multiply1/1 -> Divide4/1
  Product1/1 -> Sum/2
  Sum5/1 -> Product3/1
  [muInverse] -> Sum2/1
  Sum/1 -> Vector Concatenate2/1
  Multiply/1 -> Divide1/1
  Divide4/1 -> Sum5/2
  [muInverse] -> Sum6/1
  J/1 -> Math Function2/1
  [thetat] -> Product2/2
  Sum4/1 -> Divide3/2
  Product3/1 -> Vector Concatenate2/2
  [muInverse] -> Sum3/1
  Power/1 -> R3/1
  Switch/1 -> Math Function1/1
  Divide1/1 -> Product1/1
  [thetat] -> Divide2/1
  Constant4/1 -> Switch/3
  Sign/1 -> Product3/2
  Sum1/1 -> [thetat]
  lc/1 -> R1/1
  Product/1 -> beta1/1  "beta"
  w/1 -> Sign/1
  Sum2/1 -> Divide2/2
  Math Function2/1 -> Product/1
  Divide2/1 -> Sum/1
  Sum3/1 -> Divide1/2
  Constant1/1 -> Power/2
  Product4/1 -> Sum1/1
  theta4/1 -> Product4/1
  Square/1 -> Product7/1
  Add/1 -> Product7/2, Square/1
  Product5/1 -> Gain/1, Product7/3, Add/2
  [e] -> Product5/1
  [R] -> Product5/2
  Constant5/1 -> Product7/4
  Constant/1 -> Add/1
  Product7/1 -> [coeff1]
  [coeff1] -> Multiply/1, Divide3/1
  Constant2/1 -> Product6/1
  Constant6/1 -> Product6/2
  [CT] -> Product6/3
  [R] -> Product6/4
  [gamma] -> Product6/5
  [Nb] -> Product6/6
  [c] -> Product6/7
  [clalpha] -> Product6/8
  Constant7/1 -> Add2/1
  Gain/1 -> Add2/2
  Add2/1 -> Product6/9
  Product6/1 -> Add1/1
  Constant8/1 -> Add1/2
  Add1/1 -> [coeff2]
  [coeff2] -> Multiply1/1, Product1/2
  Arm/1 -> Bus Selector/1
  Bus Selector/1 -> [R]  "<prop4_radius_m>"
  Bus Selector/2 -> [c]  "<prop4_chord_m>"
  Bus Selector/3 -> [Nb]  "<prop4_no_of_blades>"
  Bus Selector/8 -> [theta_tip]  "<prop4_theta_tip_rad>"
  Bus Selector/7 -> [gamma]  "<prop4_lock>"
  Bus Selector/6 -> [clalpha]  "<prop4_Cl_alpha>"
  Bus Selector/5 -> [e]  "<prop4_flapping_offset_m>"
  Bus Selector/4 -> [CT]  "<prop4_ct>"
  [theta_tip] -> Product4/2

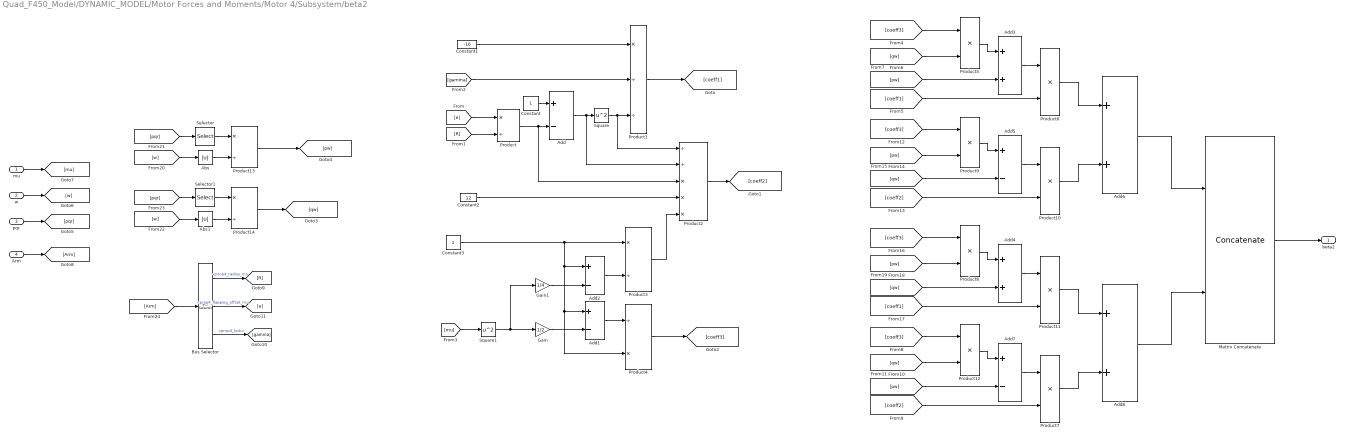
== system Quad_F450_Model/DYNAMIC_MODEL/Motor Forces and Moments/Motor 4/Subsystem/beta2 ==
  mu : Inport
  w : Inport  Port=2
  pqr : Inport  Port=3
  Arm : Inport  Port=4
  Abs : Abs  SaturateOnIntegerOverflow=off
  Abs1 : Abs  SaturateOnIntegerOverflow=off
  Add{,1..2,5,7} (5 alike) : Sum  Inputs=+-
  Add{3..4,6,8} (4 alike) : Sum
  Bus Selector : BusSelector  OutputSignals=prop4_radius_m,prop4_flapping_offset_m,prop4_lock
  Constant : Constant
  Constant1 : Constant  Value=-16
  Constant2 : Constant  Value=12
  Constant3 : Constant
  Gain : Gain  Gain=1/2
  Gain1 : Gain  Gain=1/4
  Matrix Concatenate : Concatenate  ConcatenateDimension=2
  Product{,3,13..14} (4 alike) : Product  Inputs=*/
  Product1 : Product  Inputs=*//
  Product{5..12} (8 alike) : Product
  Product2 : Product  Inputs=//***
  Product4 : Product  Inputs=/*
  Selector : Selector  InputPortWidth=3  IndexOptions=Index vector (dialog)  Indices=1  OutputSizes=1
  Selector1 : Selector  InputPortWidth=3  IndexOptions=Index vector (dialog)  Indices=1  OutputSizes=1
  Square : Math  Operator=square
  Square1 : Math  Operator=square
  beta2 : Outport
  wires:
  w/1 -> [w]
  mu/1 -> [mu]
  [e] -> Product/1
  [R] -> Product/2
  Constant/1 -> Add/1
  Product/1 -> Product2/3, Add/2
  Add/1 -> Product2/2, Square/1
  Square/1 -> Product2/1, Product1/3
  [gamma] -> Product1/2
  Constant1/1 -> Product1/1
  Constant2/1 -> Product2/4
  Constant3/1 -> Product4/2, Add1/1, Add2/1, Product3/1
  [mu] -> Square1/1
  Square1/1 -> Gain/1, Gain1/1
  Gain/1 -> Add1/2
  Gain1/1 -> Add2/2
  Add2/1 -> Product3/2
  Add1/1 -> Product4/1
  Product3/1 -> Product2/5
  Product1/1 -> [coeff1]
  Product2/1 -> [coeff2]
  Product4/1 -> [coeff3]
  [coeff3] -> Product5/1
  Product5/1 -> Add3/1
  Add3/1 -> Product6/1
  [coeff1] -> Product6/2
  [qw] -> Product5/2
  [pw] -> Add3/2
  Product6/1 -> Add6/1
  Product9/1 -> Add5/1
  [pw] -> Product9/2
  Add5/1 -> Product10/1
  [coeff2] -> Product10/2
  [qw] -> Add5/2
  [coeff3] -> Product9/1
  Product10/1 -> Add6/2
  Product12/1 -> Add7/1
  [coeff2] -> Product7/2
  [qw] -> Product12/2
  Add7/1 -> Product7/1
  Product8/1 -> Add4/1
  [coeff3] -> Product12/1
  [pw] -> Product8/2
  [pw] -> Add7/2
  Product7/1 -> Add8/2
  Add4/1 -> Product11/1
  [coeff1] -> Product11/2
  [qw] -> Add4/2
  [coeff3] -> Product8/1
  Product11/1 -> Add8/1
  Add6/1 -> Matrix Concatenate/1
  Add8/1 -> Matrix Concatenate/2
  pqr/1 -> [pqr]
  [pqr] -> Selector/1
  [w] -> Abs/1
  Selector/1 -> Product13/1
  Abs/1 -> Product13/2
  Product13/1 -> [pw]
  Abs1/1 -> Product14/2
  [w] -> Abs1/1
  Selector1/1 -> Product14/1
  Product14/1 -> [qw]
  [pqr] -> Selector1/1
  Arm/1 -> [Arm]
  [Arm] -> Bus Selector/1
  Matrix Concatenate/1 -> beta2/1
  Bus Selector/1 -> [R]  "<prop4_radius_m>"
  Bus Selector/2 -> [e]  "<prop4_flapping_offset_m>"
  Bus Selector/3 -> [gamma]  "<prop4_lock>"

== system Quad_F450_Model/DYNAMIC_MODEL/Motor Forces and Moments/Motor 4/Subsystem/lc and mu ==
  Vr : Inport
  w : Inport  Port=2
  Arm : Inport  Port=3
  Abs : Abs  SaturateOnIntegerOverflow=off
  Bus Selector : BusSelector  OutputSignals=prop4_radius_m
  Complex to Real-Imag : ComplexToRealImag  Output=Real
  Divide : Product  Inputs=*/
  Divide1 : Product  Inputs=*/
  Math Function : Math  Operator=square  SignedPower=on
  Product : Product
  Selector : Selector  InputPortWidth=3  IndexOptions=Index vector (dialog)  Indices=[1 2]  OutputSizes=1
  Selector1 : Selector  InputPortWidth=3  IndexOptions=Index vector (dialog)  Indices=[3]  OutputSizes=1
  Sqrt : Sqrt  OutputSignalType=complex
  Sum of Elements : Sum  Inputs=+
  lc : Outport
  mu : Outport  Port=2
  wires:
  Selector/1 -> Math Function/1
  Sqrt/1 -> Complex to Real-Imag/1
  Math Function/1 -> Sum of Elements/1
  w/1 -> Abs/1
  Selector1/1 -> Divide1/1
  Product/1 -> Divide/2, Divide1/2
  Divide1/1 -> lc/1  "lc"
  Vr/1 -> Selector/1, Selector1/1
  Sum of Elements/1 -> Sqrt/1
  Divide/1 -> mu/1  "mu"
  Complex to Real-Imag/1 -> Divide/1
  Abs/1 -> Product/1
  Arm/1 -> Bus Selector/1  "r"
  Bus Selector/1 -> Product/2  "<prop4_radius_m>"
